simulink model "RimlessWheelStateflowPlant"  (Simulink 7.6)
settings: Solver=ode45  StartTime=0.0  StopTime=10.0  RelTol=1e-3
libraries: simulink x1
settings Model: Creator=russt  LastModifiedBy=russt

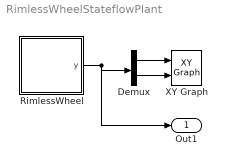
== system RimlessWheelStateflowPlant ==
  Demux : Demux  Outputs=2
  RimlessWheel : Stateflow chart  TreatAsAtomicUnit=on
  XY Graph : simulink/Sinks/XY Graph  SystemSampleTime=-1  xmin=-.5  xmax=.75  ymin=-.5  ymax=2  st=-1
  Out1 : Outport
  wires:
  RimlessWheel/1(y) -> Demux/1, Out1/1
  Demux/1 -> XY Graph/1
  Demux/2 -> XY Graph/2

== stateflow chart RimlessWheel ==
  settings: updateMethod=CONTINUOUS
  state Stance
    during:
    //derivatives
    theta_dot = thetadot;
    thetadot_dot = 9.8*sin(theta);
    //outputs
    y[0] = theta;
    y[1] = thetadot;
  (default) -> Stance : {theta=.1;thetadot=0;}
  Stance -> Stance [order 1] : [theta >= gamma + alpha]
      | {
      |   theta = gamma - alpha;
      |   thetadot = cos(2*alpha)*thetadot;
      | }
  Stance -> Stance [order 2] : [theta<=gamma-alpha]
      | {
      |   theta = gamma+alpha;
      |   thetadot = cos(2*alpha)*thetadot;
      | }
  data: theta local double; thetadot local double; y output double size=2; gamma constant double =0.08; alpha constant double =pi/8
  data theta settings: updateMethod=SF_CONTINUOUS_TIME_DATA
  data thetadot settings: updateMethod=SF_CONTINUOUS_TIME_DATA
